simulink model "center_tapped_thristor"  (R2022a)
settings: Solver=VariableStepAuto  StartTime=0.0  StopTime=0.1  RelTol=1e-3
libraries: spsGroundLib x3, spsVoltageMeasurementLib x3, spsThyristorLib x2, spsACVoltageSourceLib x1, spsCurrentMeasurementLib x1, spsLinearTransformerLib x1, spsParallelRLCBranchLib x1, spspowerguiLib x1
settings Model: Creator=P.O.M.G  LastModifiedBy=P.O.M.G

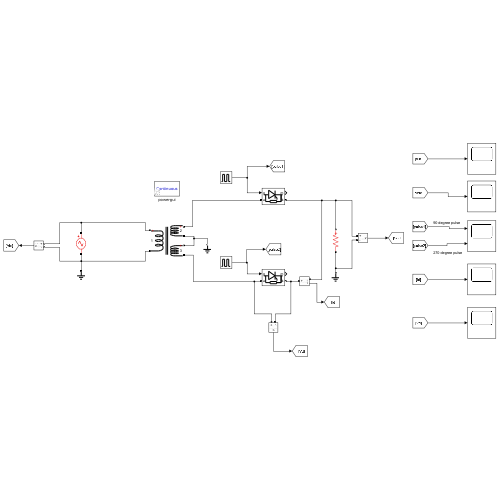
[thumbnail: Simulink's stored preview of the top-level diagram]
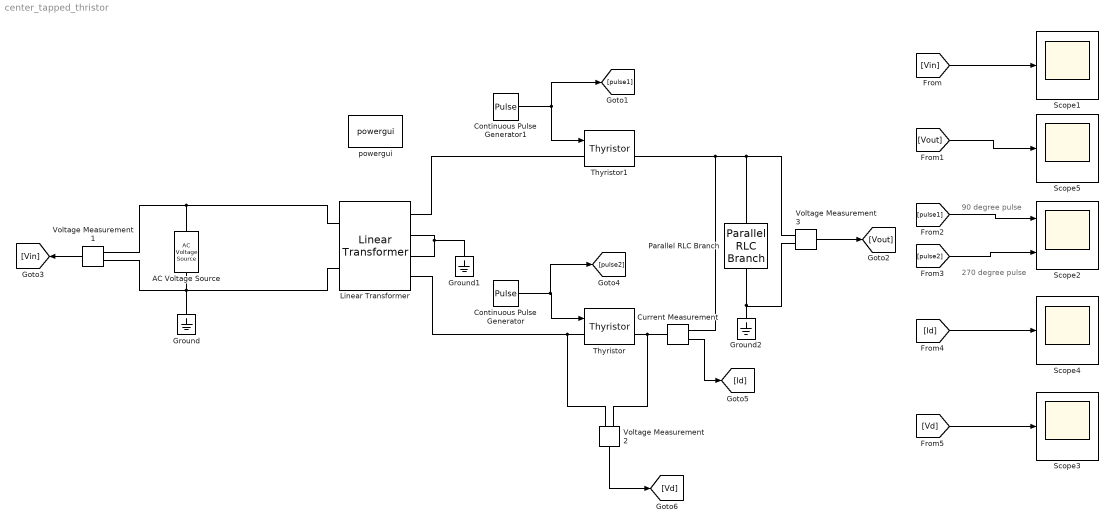
== system center_tapped_thristor ==
  note: 270 degree pulse
  note: 90 degree pulse
  AC Voltage Source : spsACVoltageSourceLib/AC Voltage Source  Amplitude=308  Phase=0  Frequency=50  SampleTime=1e-5  Measurements=None  BusType=swing  Pref=10e3  Qref=0  Qmin=-inf  Qmax=+inf
  Continuous Pulse Generator : DiscretePulseGenerator  PulseType=Time based  Period=0.02  PulseWidth=5  PhaseDelay=0.015
  Continuous Pulse Generator1 : DiscretePulseGenerator  PulseType=Time based  Period=0.02  PulseWidth=5  PhaseDelay=.005
  Current Measurement : spsCurrentMeasurementLib/Current Measurement  PhasorSimulation=off  OutputType=Complex  PSBequivalent=0
  Ground : spsGroundLib/Ground  LConnTagsString=a
  Ground1 : spsGroundLib/Ground  LConnTagsString=a
  Ground2 : spsGroundLib/Ground  LConnTagsString=a
  Linear Transformer : spsLinearTransformerLib/Linear Transformer  UNITS=pu  NominalPower=[ 250e6 60 ]  winding1=[308 0.002 0.08]  winding2=[308 0.002 0.08]  ThreeWindings=on  winding3=[308 0.002 0.08]  RmLm=[500 500]  Measurements=None  DataType=off
  Parallel RLC Branch : spsParallelRLCBranchLib/Parallel RLC Branch  LConnTagsString=a  RConnTagsString=__new0  BranchType=R  Resistance=100  Inductance=0  SetiL0=off  InitialCurrent=0  Capacitance=0  Setx0=off  InitialVoltage=0  Measurements=None
  Scope{1,3..5} (4 alike) : Scope
  Scope2 : Scope  NumInputPorts=2
  Thyristor : spsThyristorLib/Thyristor  Ron=0.001  Lon=0  Vf=0.8  IC=0  Rs=500  Cs=250e-9  Measurements=on
  Thyristor1 : spsThyristorLib/Thyristor  Ron=0.001  Lon=0  Vf=0.8  IC=0  Rs=500  Cs=250e-9  Measurements=on
  Voltage Measurement1 : spsVoltageMeasurementLib/Voltage Measurement  PhasorSimulation=off  OutputType=Complex  PSBequivalent=0
  Voltage Measurement2 : spsVoltageMeasurementLib/Voltage Measurement  PhasorSimulation=off  OutputType=Complex  PSBequivalent=0
  Voltage Measurement3 : spsVoltageMeasurementLib/Voltage Measurement  PhasorSimulation=off  OutputType=Complex  PSBequivalent=0
  powergui : spspowerguiLib/powergui  Priority=1  SimulationMode=Continuous  SampleTime=50e-6  frequency=60  Iterations=50  frequencyindice=50  Pbase=100e6  ErrMax=1e-4  UnitsV=kV  UnitsW=MW  buscounter=0  FunctionMessages=off  echomessages=off  EnableUseOfTLC=off  CurrentSourceSwitches=on  DisableSnubberDevices=off  DisableRonSwitches=off  DisableVfSwitches=off  DisplayEquations=off  AutomaticDiscreteSolvers=off  SolverType=Tustin/Backward Euler (TBE)  Interpol=off  ExternalGateDelay=off  methode=off  Ts=100  x0status=blocks  SPID=off  SwTol=0  HookPort=off  NonlinearTolerance=1e-4  nMaxIteration=100  ContinueOnMaxIteration=off  RestoreLinks=warning  ResistiveCurrentMeasurement=off  Frange=[0:2:500]  Ylog=off  Xlog=on  ShowGrid=off  save=off  variable=ZData  structure=0  ZoomFFT=off  StartTime=0.0  cycles=1  DisplayStyle=1  fundamental=60  FreqAxis=off  MaxFrequency=1000  frequencyindicesteady=1  RmsSteady=1  display=off
  wires:
  Voltage Measurement1/1 -> [Vin]
  Continuous Pulse Generator/1 -> [pulse2], Thyristor/1
  Continuous Pulse Generator1/1 -> [pulse1], Thyristor1/1
  Voltage Measurement3/1 -> [Vout]
  [Vout] -> Scope5/1
  Current Measurement/1 -> [Id]
  Voltage Measurement2/1 -> [Vd]
  [Id] -> Scope4/1
  [pulse2] -> Scope2/2
  [pulse1] -> Scope2/1
  [Vd] -> Scope3/1
  [Vin] -> Scope1/1
  connections:
  Ground/LConn1 -- Linear Transformer/LConn2 -- Voltage Measurement1/LConn2 -- AC Voltage Source/LConn1
  Voltage Measurement1/LConn1 -- AC Voltage Source/RConn1 -- Linear Transformer/LConn1
  Linear Transformer/RConn2 -- Ground1/LConn1 -- Linear Transformer/RConn3
  Thyristor1/LConn1 -- Linear Transformer/RConn1
  Thyristor/LConn1 -- Voltage Measurement2/LConn1 -- Linear Transformer/RConn4
  Parallel RLC Branch/LConn1 -- Voltage Measurement3/LConn1 -- Current Measurement/RConn1 -- Thyristor1/RConn1
  Ground2/LConn1 -- Parallel RLC Branch/RConn1 -- Voltage Measurement3/LConn2
  Current Measurement/LConn1 -- Voltage Measurement2/LConn2 -- Thyristor/RConn1
